simulink model "controllore_sim"  (Simulink 8.3)
settings: Solver=ode45  StartTime=0.0  StopTime=20  RelTol=1e-3
values from neighbouring files (symbols this model uses):
  D1 = 1    [controllore.m]
  D2 = 1    [controllore.m]
  Dp = 1    [controllore.m]
  wp = 1000    [controllore.m]
libraries: cstblocks x2, simulink x1
settings Model: Creator=matdo  LastModifiedBy=matdo
settings DataIOCC: SignalLoggingSaveFormat=Dataset
settings DebuggingCC: UnderspecifiedInitializationDetection=Simplified  StateNameClashWarn=none
settings GRTTargetCC: CombineOutputUpdateFcns=on  GRTInterface=off

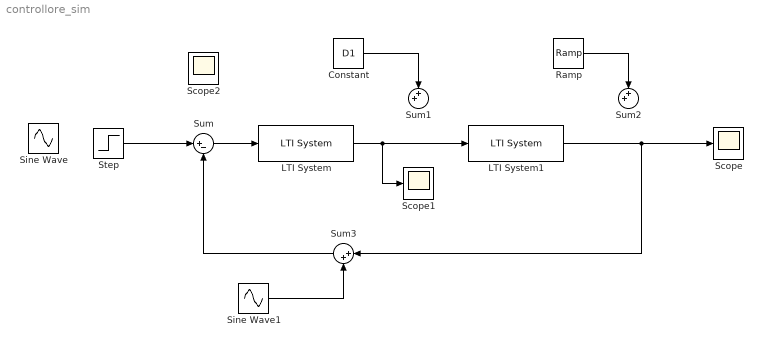
== system controllore_sim ==
  Constant : Constant  Value=D1
  LTI System : cstblocks/LTI System  sys=Ci  IC=[]
  LTI System1 : cstblocks/LTI System  sys=F  IC=[]
  Ramp : simulink/Sources/Ramp  slope=D2  start=0  X0=0
  Scope : Scope
  Scope1 : Scope
  Scope2 : Scope
      settings: SaveName=ScopeData2
  Sine Wave : Sin  Frequency=0.5  SampleTime=0
  Sine Wave1 : Sin  Amplitude=Dp  Frequency=wp  SampleTime=0
  Step : Step  Time=0  SampleTime=0
  Sum : Sum  Inputs=|+-
  Sum1 : Sum  Inputs=++|
  Sum2 : Sum  Inputs=++|
  Sum3 : Sum  Inputs=|++
  wires:
  Sine Wave1/1 -> Sum3/2
  Constant/1 -> Sum1/1
  Ramp/1 -> Sum2/1
  LTI System/1 -> Scope1/1, LTI System1/1
  LTI System1/1 -> Sum3/1, Scope/1
  Sum/1 -> LTI System/1
  Sum3/1 -> Sum/2
  Step/1 -> Sum/1
